simulink model "openloop_FOC"  (R2024b)
settings: Solver=VariableStepAuto  StartTime=0.0  StopTime=8  MaxStep=0.00001  RelTol=1e-3
libraries: simulink x1
settings Model: Creator=27abd  LastModifiedBy=27abd

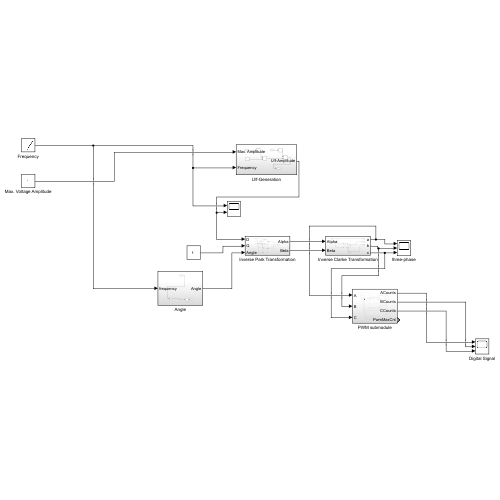
[thumbnail: Simulink's stored preview of the top-level diagram]
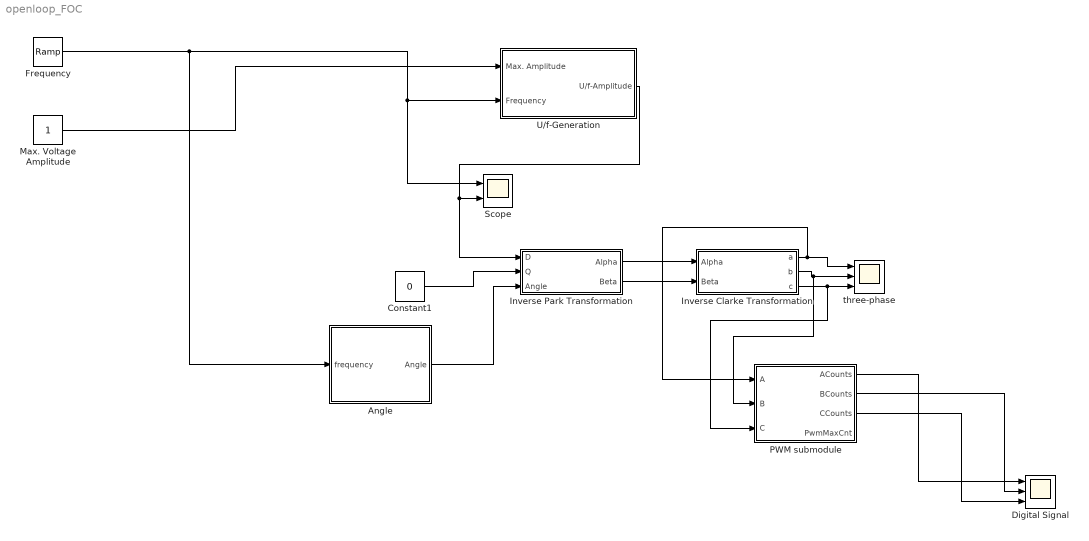
== system openloop_FOC ==
  Angle : Subsystem
  Constant1 : Constant  Value=0
  Digital Signal : Scope  NumInputPorts=3
  Frequency : simulink/Sources/Ramp  slope=10  start=0  InitialOutput=-10
  Inverse Clarke Transformation : Subsystem
  Inverse Park Transformation : Subsystem
  Max. Voltage Amplitude : Constant
  PWM submodule : Subsystem
  Scope : Scope  NumInputPorts=2
  U/f-Generation : Subsystem
  three-phase : Scope  NumInputPorts=3
  wires:
  Frequency/1 -> Angle/1(frequency), Scope/1, U/f-Generation/2(Frequency)
  Max. Voltage Amplitude/1 -> U/f-Generation/1(Max. Amplitude)
  U/f-Generation/1(U/f-Amplitude) -> Inverse Park Transformation/1(D), Scope/2
  Constant1/1 -> Inverse Park Transformation/2(Q)
  Angle/1(Angle) -> Inverse Park Transformation/3(Angle)
  Inverse Park Transformation/1(Alpha) -> Inverse Clarke Transformation/1(Alpha)
  Inverse Park Transformation/2(Beta) -> Inverse Clarke Transformation/2(Beta)
  Inverse Clarke Transformation/1(a) -> PWM submodule/1(A), three-phase/1
  Inverse Clarke Transformation/2(b) -> PWM submodule/2(B), three-phase/2
  Inverse Clarke Transformation/3(c) -> PWM submodule/3(C), three-phase/3
  PWM submodule/1(ACounts) -> Digital Signal/1
  PWM submodule/2(BCounts) -> Digital Signal/2
  PWM submodule/3(CCounts) -> Digital Signal/3

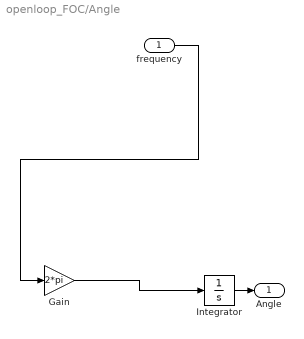
== system openloop_FOC/Angle ==
  frequency : Inport
  Gain : Gain  Gain=2*pi
  Integrator : Integrator
  Angle : Outport
  wires:
  Gain/1 -> Integrator/1
  Integrator/1 -> Angle/1
  frequency/1 -> Gain/1

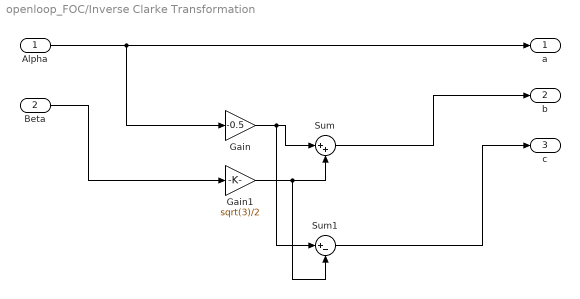
== system openloop_FOC/Inverse Clarke Transformation ==
  Alpha : Inport
  Beta : Inport  Port=2
  Gain : Gain  Gain=-0.5
  Gain1 : Gain  Gain=sqrt(3)/2
  Sum : Sum  Inputs=|++
  Sum1 : Sum  Inputs=|+-
  a : Outport
  b : Outport  Port=2
  c : Outport  Port=3
  wires:
  Alpha/1 -> Gain/1, a/1
  Beta/1 -> Gain1/1
  Gain/1 -> Sum1/1, Sum/1
  Gain1/1 -> Sum1/2, Sum/2
  Sum/1 -> b/1
  Sum1/1 -> c/1

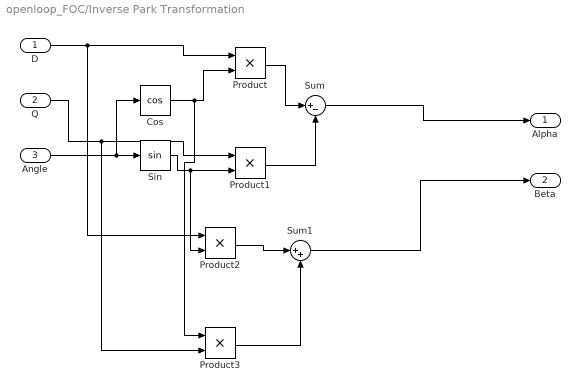
== system openloop_FOC/Inverse Park Transformation ==
  D : Inport
  Q : Inport  Port=2
  Angle : Inport  Port=3
  Cos : Trigonometry  Operator=cos
  Product{,1..3} (4 alike) : Product
  Sin : Trigonometry
  Sum : Sum  Inputs=|+-
  Sum1 : Sum  Inputs=|++
  Alpha : Outport
  Beta : Outport  Port=2
  wires:
  Angle/1 -> Cos/1, Sin/1
  D/1 -> Product2/1, Product/1
  Cos/1 -> Product3/1, Product/2
  Q/1 -> Product3/2, Product1/1
  Sin/1 -> Product2/2, Product1/2
  Product1/1 -> Sum/2
  Product/1 -> Sum/1
  Sum/1 -> Alpha/1
  Sum1/1 -> Beta/1
  Product2/1 -> Sum1/1
  Product3/1 -> Sum1/2

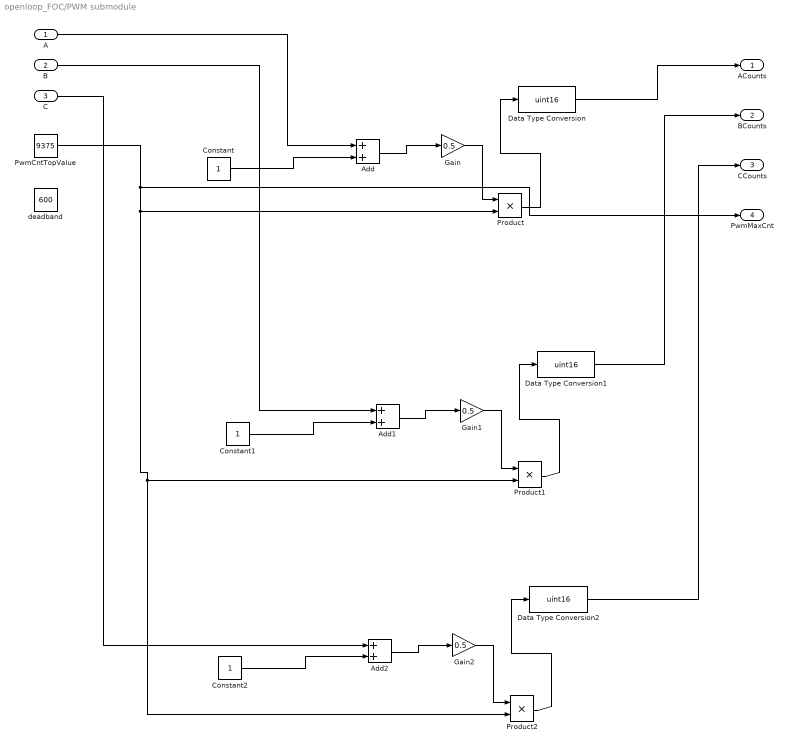
== system openloop_FOC/PWM submodule ==
  A : Inport
  B : Inport  Port=2
  C : Inport  Port=3
  Add : Sum
  Add1 : Sum
  Add2 : Sum
  Constant : Constant
  Constant1 : Constant
  Constant2 : Constant
  Data Type Conversion : DataTypeConversion  OutDataTypeStr=uint16  SaturateOnIntegerOverflow=off  RndMeth=Floor
  Data Type Conversion1 : DataTypeConversion  OutDataTypeStr=uint16  SaturateOnIntegerOverflow=off  RndMeth=Floor
  Data Type Conversion2 : DataTypeConversion  OutDataTypeStr=uint16  SaturateOnIntegerOverflow=off  RndMeth=Floor
  Gain : Gain  Gain=0.5
  Gain1 : Gain  Gain=0.5
  Gain2 : Gain  Gain=0.5
  Product : Product
  Product1 : Product
  Product2 : Product
  PwmCntTopValue : Constant  Value=9375
  deadband : Constant  Value=600
  ACounts : Outport
  BCounts : Outport  Port=2
  CCounts : Outport  Port=3
  PwmMaxCnt : Outport  Port=4
  wires:
  A/1 -> Add/1
  Constant/1 -> Add/2
  Add/1 -> Gain/1
  Gain/1 -> Product/1
  PwmCntTopValue/1 -> PwmMaxCnt/1, Product2/2, Product1/2, Product/2
  Product/1 -> Data Type Conversion/1
  Product1/1 -> Data Type Conversion1/1
  Constant1/1 -> Add1/2
  B/1 -> Add1/1
  Gain1/1 -> Product1/1
  Add1/1 -> Gain1/1
  Gain2/1 -> Product2/1
  Product2/1 -> Data Type Conversion2/1
  Constant2/1 -> Add2/2
  Add2/1 -> Gain2/1
  C/1 -> Add2/1
  Data Type Conversion/1 -> ACounts/1
  Data Type Conversion1/1 -> BCounts/1
  Data Type Conversion2/1 -> CCounts/1

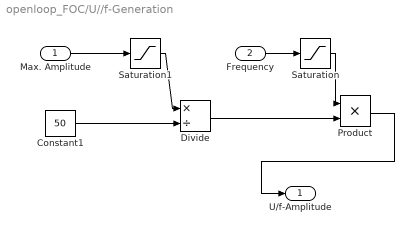
== system openloop_FOC/U//f-Generation ==
  Max. Amplitude : Inport
  Frequency : Inport  Port=2
  Constant1 : Constant  Value=50
  Divide : Product  Inputs=*/
  Product : Product
  Saturation : Saturate  UpperLimit=50  LowerLimit=0
  Saturation1 : Saturate  UpperLimit=100  LowerLimit=0
  U/f-Amplitude : Outport
  wires:
  Saturation/1 -> Product/1
  Max. Amplitude/1 -> Saturation1/1
  Product/1 -> U/f-Amplitude/1
  Saturation1/1 -> Divide/1
  Constant1/1 -> Divide/2
  Frequency/1 -> Saturation/1
  Divide/1 -> Product/2
